simulink model "modelo"  (R2018a)
settings: Solver=VariableStepAuto  StartTime=0.0  StopTime=10.0  RelTol=1e-3
values from neighbouring files (symbols this model uses):
  A = [1  -0.49  -0.495]    [ativ1q2t2.m]    (also in step_imp_ma_mf.m = [-1 1; tf_conti.m = 1)
  B = [0 0.008856 0.004428]    [ativ1q2t2.m]    (also in step_imp_ma_mf.m = [0; 1])
  C = [2 1]    [step_imp_ma_mf.m]
  D = [0]    [step_imp_ma_mf.m]
  kd = 0    [step_imp_ma_mf.m]
  ki = 0    [step_imp_ma_mf.m]
  kp = 10    [step_imp_ma_mf.m]
libraries: simulink x1
settings Model: Creator=mylen  LastModifiedBy=mylen

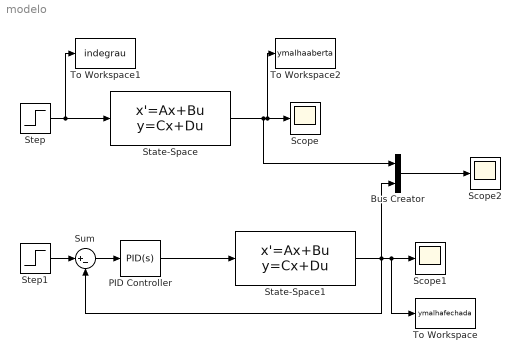
== system modelo ==
  Bus Creator : BusCreator  Inputs=2
  PID Controller : simulink/Continuous/PID Controller  Controller=PID  TimeDomain=Continuous-time  SampleTime=-1  IntegratorMethod=Forward Euler  FilterMethod=Forward Euler  Form=Parallel  UseFilter=on  ControllerParametersSource=internal  P=kp  I=ki  D=kd  N=100  InitialConditionSource=internal  InitialConditionForIntegrator=0  InitialConditionForFilter=0  ExternalReset=none  LimitOutput=off  UpperSaturationLimit=inf  LowerSaturationLimit=-inf  LinearizeAsGain=on  AntiWindupMode=none  Kb=1  TrackingMode=off  Kt=1  PParamMin=[]  PParamMax=[]  IParamMin=[]  IParamMax=[]  DParamMin=[]  DParamMax=[]  NParamMin=[]  NParamMax=[]  KbParamMin=[]  KbParamMax=[]  KtParamMin=[]  KtParamMax=[]  POutMin=[]  POutMax=[]  IOutMin=[]  IOutMax=[]  DOutMin=[]  DOutMax=[]  NOutMin=[]  NOutMax=[]  KbOutMin=[]  KbOutMax=[]  KtOutMin=[]  KtOutMax=[]  IntegratorOutMin=[]  IntegratorOutMax=[]  FilterOutMin=[]  FilterOutMax=[]  SumOutMin=[]  SumOutMax=[]  SumI1OutMin=[]  SumI1OutMax=[]  SumI2OutMin=[]  SumI2OutMax=[]  SumI3OutMin=[]  SumI3OutMax=[]  SumDOutMin=[]  SumDOutMax=[]  SaturationOutMin=[]  SaturationOutMax=[]  IntegratorContinuousStateAttributes=''  IntegratorStateMustResolveToSignalObject=off  IntegratorRTWStateStorageClass=Auto  FilterContinuousStateAttributes=''  FilterStateMustResolveToSignalObject=off  FilterRTWStateStorageClass=Auto  DifferentiatorICPrevScaledInput=0  DifferentiatorOutMin=[]  DifferentiatorOutMax=[]  FilterDiffOutCoefMin=[]  FilterDiffOutCoefMax=[]  SumDenOutMin=[]  SumDenOutMax=[]  SumNumOutMin=[]  SumNumOutMax=[]  ReciprocalOutMin=[]  ReciprocalOutMax=[]  DivideOutMin=[]  DivideOutMax=[]  TunerSelectOption=Transfer Function Based (PID Tuner App)
  Scope : Scope
  Scope1 : Scope
  Scope2 : Scope
  State-Space : StateSpace  A=A  B=B  C=C  D=D  InitialCondition=0
  State-Space1 : StateSpace  A=A  B=B  C=C  D=D  InitialCondition=0
  Step : Step  Time=0  SampleTime=0
  Step1 : Step  Time=0  SampleTime=0
  Sum : Sum  Inputs=|+-
  To Workspace : ToWorkspace  VariableName=ymalhafechada  SampleTime=-1
  To Workspace1 : ToWorkspace  VariableName=indegrau  SampleTime=-1
  To Workspace2 : ToWorkspace  VariableName=ymalhaaberta  SampleTime=-1
  wires:
  State-Space/1 -> Bus Creator/1, To Workspace2/1, Scope/1
  Step/1 -> To Workspace1/1, State-Space/1
  Step1/1 -> Sum/1
  Sum/1 -> PID Controller/1
  PID Controller/1 -> State-Space1/1
  State-Space1/1 -> Bus Creator/2, Sum/2, To Workspace/1, Scope1/1
  Bus Creator/1 -> Scope2/1
